simulink model "Control_project_Paw"  (R2016a)
settings: Solver=VariableStepAuto  StartTime=0.0  StopTime=10.0  RelTol=1e-3
libraries: simulink x1
settings Model: Creator=User  LastModifiedBy=User

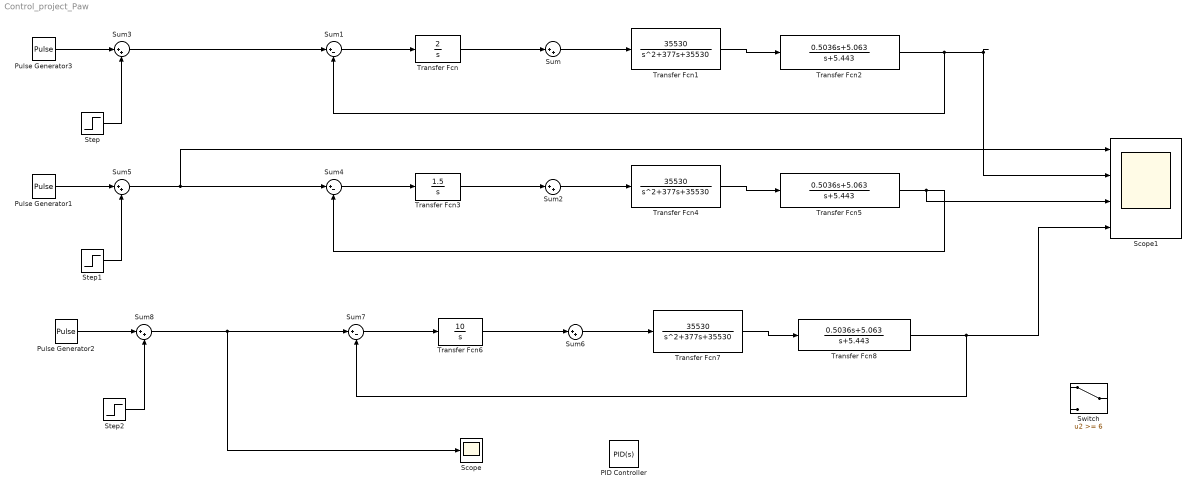
== system Control_project_Paw ==
  PID Controller : simulink/Continuous/PID Controller  Controller=PID  TimeDomain=Continuous-time  SampleTime=-1  IntegratorMethod=Forward Euler  FilterMethod=Forward Euler  Form=Parallel  UseFilter=on  ControllerParametersSource=internal  P=0  I=2  D=0  N=100  InitialConditionSource=internal  InitialConditionForIntegrator=0  InitialConditionForFilter=0  ExternalReset=none  LimitOutput=off  UpperSaturationLimit=inf  LowerSaturationLimit=-inf  LinearizeAsGain=on  AntiWindupMode=none  Kb=1  TrackingMode=off  Kt=1  PParamMin=[]  PParamMax=[]  IParamMin=[]  IParamMax=[]  DParamMin=[]  DParamMax=[]  NParamMin=[]  NParamMax=[]  KbParamMin=[]  KbParamMax=[]  KtParamMin=[]  KtParamMax=[]  POutMin=[]  POutMax=[]  IOutMin=[]  IOutMax=[]  DOutMin=[]  DOutMax=[]  NOutMin=[]  NOutMax=[]  KbOutMin=[]  KbOutMax=[]  KtOutMin=[]  KtOutMax=[]  IntegratorOutMin=[]  IntegratorOutMax=[]  FilterOutMin=[]  FilterOutMax=[]  SumOutMin=[]  SumOutMax=[]  SumI1OutMin=[]  SumI1OutMax=[]  SumI2OutMin=[]  SumI2OutMax=[]  SumI3OutMin=[]  SumI3OutMax=[]  SumDOutMin=[]  SumDOutMax=[]  SaturationOutMin=[]  SaturationOutMax=[]  IntegratorContinuousStateAttributes=''  IntegratorStateMustResolveToSignalObject=off  IntegratorRTWStateStorageClass=Auto  FilterContinuousStateAttributes=''  FilterStateMustResolveToSignalObject=off  FilterRTWStateStorageClass=Auto  DifferentiatorICPrevScaledInput=0  DifferentiatorOutMin=[]  DifferentiatorOutMax=[]
  Pulse Generator1 : DiscretePulseGenerator  PulseType=Time based  Amplitude=15  Period=8  PulseWidth=50  PhaseDelay=1
  Pulse Generator2 : DiscretePulseGenerator  PulseType=Time based  Amplitude=15  Period=8  PulseWidth=50  PhaseDelay=1
  Pulse Generator3 : DiscretePulseGenerator  PulseType=Time based  Amplitude=15  Period=8  PulseWidth=50  PhaseDelay=1
  Scope : Scope
  Scope1 : Scope  NumInputPorts=4
  Step : Step  Before=5  After=5  SampleTime=0
  Step1 : Step  Before=5  After=5  SampleTime=0
  Step2 : Step  Before=5  After=5  SampleTime=0
  Sum{,2..3,5..6,8} (6 alike) : Sum  Inputs=|++
  Sum1 : Sum  Inputs=|+-
  Sum4 : Sum  Inputs=|+-
  Sum7 : Sum  Inputs=|+-
  Switch : Switch  Threshold=6
  Transfer Fcn : TransferFcn  Numerator=[2]  Denominator=[1 0]
  Transfer Fcn1 : TransferFcn  Numerator=[35530]  Denominator="[1  377 35530]"
  Transfer Fcn2 : TransferFcn  Numerator=[0.5036 5.063]  Denominator=[1 5.443]
  Transfer Fcn3 : TransferFcn  Numerator=[1.5]  Denominator=[1 0]
  Transfer Fcn4 : TransferFcn  Numerator=[35530]  Denominator="[1  377 35530]"
  Transfer Fcn5 : TransferFcn  Numerator=[0.5036 5.063]  Denominator=[1 5.443]
  Transfer Fcn6 : TransferFcn  Numerator=[10]  Denominator=[1 0]
  Transfer Fcn7 : TransferFcn  Numerator=[35530]  Denominator="[1  377 35530]"
  Transfer Fcn8 : TransferFcn  Numerator=[0.5036 5.063]  Denominator=[1 5.443]
  wires:
  Transfer Fcn/1 -> Sum/1
  Transfer Fcn1/1 -> Transfer Fcn2/1
  Sum/1 -> Transfer Fcn1/1
  Transfer Fcn2/1 -> Scope1/2, Sum1/2
  Sum1/1 -> Transfer Fcn/1
  Pulse Generator3/1 -> Sum3/1
  Step/1 -> Sum3/2
  Sum3/1 -> Sum1/1
  Transfer Fcn3/1 -> Sum2/1
  Sum2/1 -> Transfer Fcn4/1
  Sum4/1 -> Transfer Fcn3/1
  Pulse Generator1/1 -> Sum5/1
  Step1/1 -> Sum5/2
  Sum5/1 -> Scope1/1, Sum4/1
  Transfer Fcn6/1 -> Sum6/1
  Sum6/1 -> Transfer Fcn7/1
  Sum7/1 -> Transfer Fcn6/1
  Pulse Generator2/1 -> Sum8/1
  Step2/1 -> Sum8/2
  Sum8/1 -> Scope/1, Sum7/1
  Transfer Fcn7/1 -> Transfer Fcn8/1
  Transfer Fcn4/1 -> Transfer Fcn5/1
  Transfer Fcn5/1 -> Sum4/2, Scope1/3
  Transfer Fcn8/1 -> Sum7/2, Scope1/4
